simulink model "bebop_vert"  (R2019b)
settings: Solver=VariableStepAuto  StartTime=0.0  StopTime=30  RelTol=1e-3
values from neighbouring files (symbols this model uses):
  c = 2 * sqrt(k*m2) * 0.8    [MatToSimulink_test_tutorial.m]
  deltax0 = 0.025    [MatToSimulink_test_tutorial.m]
  g = 9.81    [MatToSimulink_test_tutorial.m]
  h_des = 2    [MatToSimulink_test_tutorial.m]
  k = 1.1 * m2 *g / (deltax0 * 0.2)    (= 431.64)    [MatToSimulink_test_tutorial.m]
  m1 = 0.3    [MatToSimulink_test_tutorial.m]
  m2 = 0.2    [MatToSimulink_test_tutorial.m]
  omega_motor = 50    [MatToSimulink_test_tutorial.m]
  x1_0 = 0    [MatToSimulink_test_tutorial.m]
  x2_0 = deltax0 - m2*g/k    (= 0.0204545454545)    [MatToSimulink_test_tutorial.m]
libraries: simulink x1
settings Model: Creator=ASUS  LastModifiedBy=ASUS

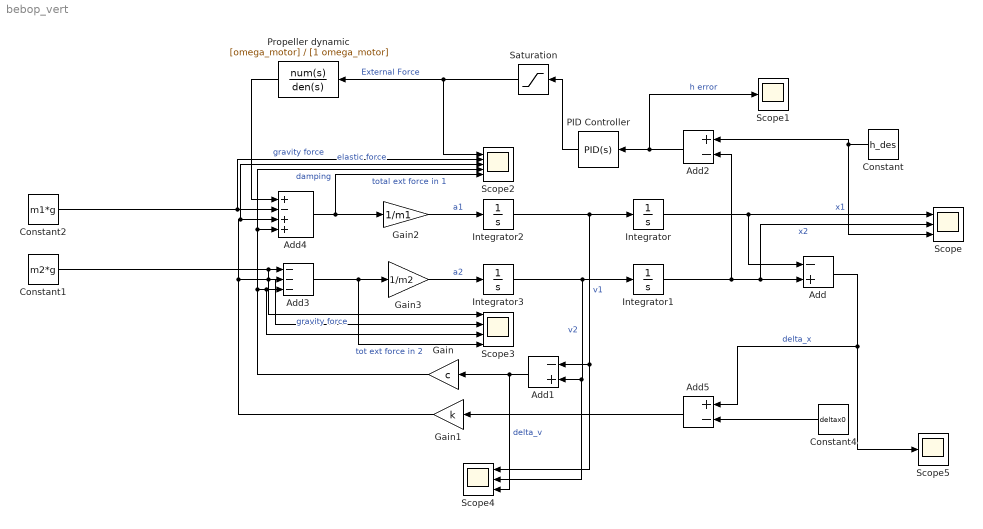
== system bebop_vert ==
  Add : Sum  Inputs=-+
  Add1 : Sum  Inputs=-+
  Add2 : Sum  Inputs=+-
  Add3 : Sum  Inputs=---
  Add4 : Sum  Inputs=+-++
  Add5 : Sum  Inputs=+-
  Constant : Constant  Value=h_des
  Constant1 : Constant  Value=m2*g
  Constant2 : Constant  Value=m1*g
  Constant4 : Constant  Value=deltax0
  Gain : Gain  Gain=c
  Gain1 : Gain  Gain=k
  Gain2 : Gain  Gain=1/m1
  Gain3 : Gain  Gain=1/m2
  Integrator : Integrator  InitialCondition=x1_0
  Integrator1 : Integrator  InitialCondition=x2_0
  Integrator2 : Integrator
  Integrator3 : Integrator
  PID Controller : simulink/Continuous/PID Controller  Controller=PID  Form=Parallel  TimeDomain=Continuous-time  SampleTime=-1  IntegratorMethod=Forward Euler  FilterMethod=Forward Euler  ControllerParametersSource=internal  P=10  I=0  D=1  UseFilter=on  N=100  TunerSelectOption=Transfer Function Based (PID Tuner App)  InitialConditionSource=internal  InitialConditionForIntegrator=0  InitialConditionForFilter=0  DifferentiatorICPrevScaledInput=0  ExternalReset=none  TrackingMode=off  Kt=1  LimitOutput=off  UpperSaturationLimit=inf  LowerSaturationLimit=-inf  LinearizeAsGain=on  AntiWindupMode=none  Kb=1  POutMin=[]  POutMax=[]  IOutMin=[]  IOutMax=[]  DOutMin=[]  DOutMax=[]  NOutMin=[]  NOutMax=[]  SumOutMin=[]  SumOutMax=[]  SaturationOutMin=[]  SaturationOutMax=[]  PParamMin=[]  PParamMax=[]  IParamMin=[]  IParamMax=[]  DParamMin=[]  DParamMax=[]  NParamMin=[]  NParamMax=[]  KbParamMin=[]  KbParamMax=[]  KtParamMin=[]  KtParamMax=[]  KbOutMin=[]  KbOutMax=[]  KtOutMin=[]  KtOutMax=[]  IntegratorOutMin=[]  IntegratorOutMax=[]  FilterOutMin=[]  FilterOutMax=[]  SumI1OutMin=[]  SumI1OutMax=[]  SumI2OutMin=[]  SumI2OutMax=[]  SumI3OutMin=[]  SumI3OutMax=[]  SumI4OutMin=[]  SumI4OutMax=[]  SumDOutMin=[]  SumDOutMax=[]  DifferentiatorOutMin=[]  DifferentiatorOutMax=[]  FilterDiffOutCoefMin=[]  FilterDiffOutCoefMax=[]  ReciprocalOutMin=[]  ReciprocalOutMax=[]  SumDenOutMin=[]  SumDenOutMax=[]  SumNumOutMin=[]  SumNumOutMax=[]  DivideOutMin=[]  DivideOutMax=[]  IntegratorContinuousStateAttributes=''  IntegratorStateMustResolveToSignalObject=off  IntegratorRTWStateStorageClass=Auto  FilterContinuousStateAttributes=''  FilterStateMustResolveToSignalObject=off  FilterRTWStateStorageClass=Auto  ParallelPVariant=InternalParameters  IdealPVariant=Disabled  IVariant=InternalParameters  DVariant=InternalParameters  IntegratorVariant=Continuous  SatVariant=Disabled  AWVariant=Passthrough  PCopyVariant=Disabled  TRVariant=Disabled  FdbkBlocksVariant=Forward  IdealPFdbkVariant=Disabled  SatFdbkVariant=Disabled  DerivativeFilterVariant=ContFilter  NVariant=InternalParameters  NCopyVariant=Disabled  FilterICVariant=InternalICsFilter  IntegratorICVariant=InternalICs  ExternalResetVariant=Disabled  TRSumVariant=Passthrough  SumFdbkVariant=Disabled  SumVariant=Sum_PID
  Propeller dynamic : TransferFcn  Numerator=[omega_motor]  Denominator=[1 omega_motor]
  Saturation : Saturate  UpperLimit=50  LowerLimit=0
  Scope : Scope  NumInputPorts=3
  Scope1 : Scope
  Scope2 : Scope  NumInputPorts=5
  Scope3 : Scope  NumInputPorts=4
  Scope4 : Scope  NumInputPorts=3
  Scope5 : Scope
  wires:
  Integrator2/1 -> Scope4/1, Add1/1, Integrator/1  "v1"
  Integrator3/1 -> Scope4/2, Add1/2, Integrator1/1  "v2"
  Integrator1/1 -> Add2/2, Scope/2, Add/2  "x2"
  Integrator/1 -> Scope/1, Add/1  "x1"
  Gain2/1 -> Integrator2/1  "a1"
  Gain3/1 -> Integrator3/1  "a2"
  Add/1 -> Add5/1, Scope5/1  "delta_x"
  Add1/1 -> Scope4/3, Gain/1  "delta_v"
  Constant/1 -> Add2/1, Scope/3
  Add2/1 -> Scope1/1, PID Controller/1  "h error"
  PID Controller/1 -> Saturation/1
  Gain1/1 -> Scope2/3, Add4/3, Scope3/2, Add3/2  "elastic force"
  Gain/1 -> Scope2/4, Add4/4, Scope3/3, Add3/3  "damping"
  Constant1/1 -> Scope3/1, Add3/1  "gravity force"
  Add3/1 -> Scope3/4, Gain3/1  "tot ext force in 2"
  Add4/1 -> Scope2/5, Gain2/1  "total ext force in 1"
  Constant2/1 -> Scope2/2, Add4/2  "gravity force"
  Constant4/1 -> Add5/2
  Add5/1 -> Gain1/1
  Saturation/1 -> Scope2/1, Propeller dynamic/1  "External Force"
  Propeller dynamic/1 -> Add4/1
